simulink model "BitwiseOperator_TestGen12"  (R2017b)
settings: Solver=FixedStepDiscrete  StartTime=0.0  StopTime=10.0  RelTol=1e-3
undefined symbols (not defined in the file): Block_TestLib, enable
libraries: simulink x1
settings Model: Creator=hbourbou  LastModifiedBy=hbourbou
settings DebuggingCC: ParameterOverflowMsg=none

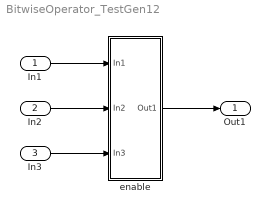
== system BitwiseOperator_TestGen12 ==
  In1 : Inport
  In2 : Inport  Port=2
  In3 : Inport  Port=3
  enable : Subsystem  AncestorBlock=Block_TestLib/enable
  Out1 : Outport
  wires:
  In1/1 -> enable/1(In1)
  In2/1 -> enable/2(In2)
  In3/1 -> enable/3(In3)
  enable/1(Out1) -> Out1/1

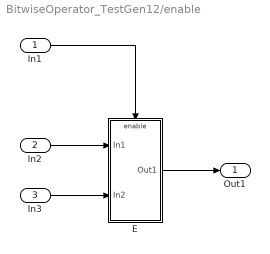
== system BitwiseOperator_TestGen12/enable ==
  In1 : Inport  OutDataTypeStr=boolean
  In2 : Inport  Port=2
  In3 : Inport  Port=3
  E : Subsystem  TreatAsAtomicUnit=on
  Out1 : Outport
  wires:
  In1/1 -> E/Enable
  In2/1 -> E/1(In1)
  In3/1 -> E/2(In2)
  E/1(Out1) -> Out1/1

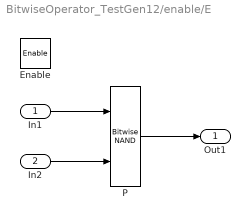
== system BitwiseOperator_TestGen12/enable/E ==
  In1 : Inport  OutDataTypeStr=uint16  PortDimensions=[2 3]
  In2 : Inport  Port=2
  Enable : EnablePort
  P : simulink/Logic and Bit Operations/Bitwise Operator  logicop=NAND  UseBitMask=off  NumInputPorts=2  BitMask=bin2dec('11011001')  BitMaskRealWorld=Stored Integer
  Out1 : Outport
  wires:
  In1/1 -> P/1
  In2/1 -> P/2
  P/1 -> Out1/1
